simulink model "encoder"  (R2022b)
settings: Solver=VariableStepAuto  StartTime=0.0  StopTime=10.0  RelTol=1e-3
libraries: simulink x1, spsSampleandHoldLib x1
settings Model: Creator=mluser  LastModifiedBy=mluser

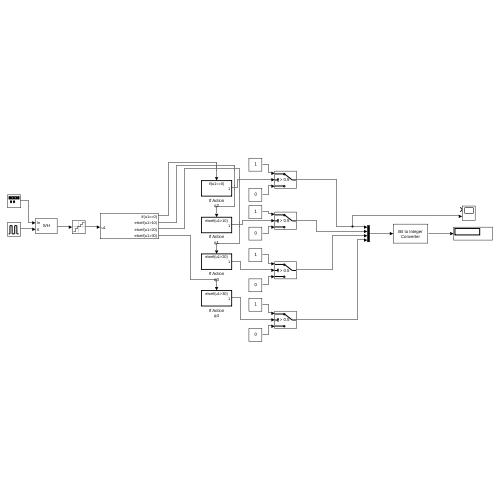
[thumbnail: Simulink's stored preview of the top-level diagram]
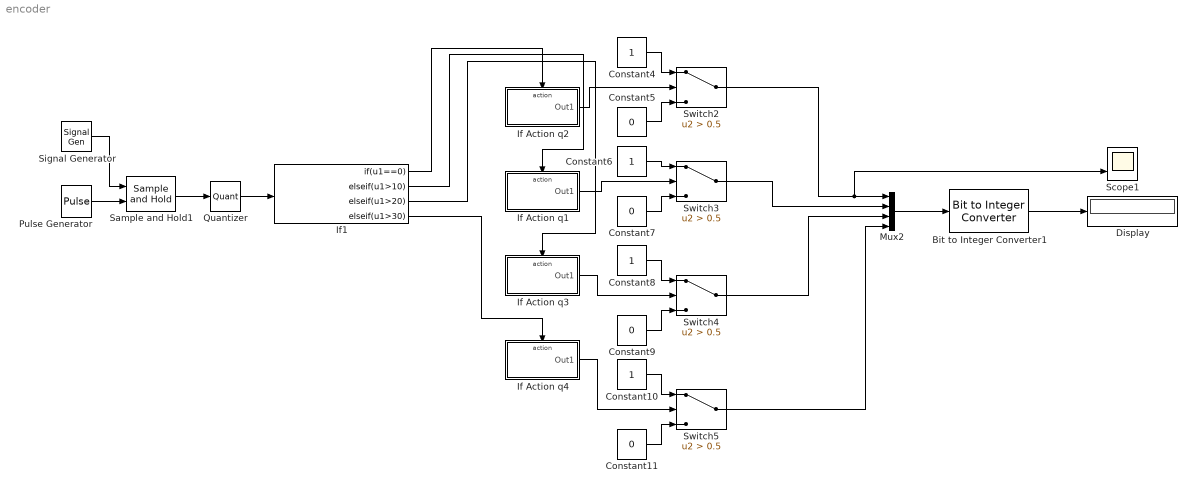
== system encoder ==
  Bit to Integer Converter1 : simulink/Logic and Bit Operations/Bit to Integer Converter  nbits=4  bitOrder=MSB first  signedOutputValues=Unsigned  outDtype=Inherit via internal rule  outDtypeSigned=Inherit via internal rule
  Constant{4,6,8,10} (4 alike) : Constant
  Constant{5,7,9,11} (4 alike) : Constant  Value=0
  Display : Display
  If Action q1 : Subsystem  TreatAsAtomicUnit=on
  If Action q2 : Subsystem  TreatAsAtomicUnit=on
  If Action q3 : Subsystem  TreatAsAtomicUnit=on
  If Action q4 : Subsystem  TreatAsAtomicUnit=on
  If1 : If  IfExpression=u1==0  ElseIfExpressions=u1>10,u1>20,u1>30  ShowElse=off
  Mux2 : Mux
  Pulse Generator : DiscretePulseGenerator  PulseType=Time based  Period=0.1  PulseWidth=5
  Quantizer : Quantizer
  Sample and Hold1 : spsSampleandHoldLib/Sample and Hold  ic=0  Ts=0
      settings: LibrarySourceBlock=|
      | sps_lib/Control/Sample and
      | Hold
  Scope1 : Scope  NumInputPorts=2
  Signal Generator : SignalGenerator  Amplitude=40  Units=rad/sec
  Switch{2..5} (4 alike) : Switch  Criteria=u2 > Threshold  Threshold=0.5  SaturateOnIntegerOverflow=off  InputSameDT=off
  wires:
  Pulse Generator/1 -> Sample and Hold1/2
  Signal Generator/1 -> Sample and Hold1/1
  Bit to Integer Converter1/1 -> Display/1
  If1/1 -> If Action q2/Action
  If1/2 -> If Action q1/Action
  If1/3 -> If Action q3/Action
  Mux2/1 -> Bit to Integer Converter1/1
  If1/4 -> If Action q4/Action
  Switch2/1 -> Scope1/2, Mux2/1
  Constant5/1 -> Switch2/3
  If Action q2/1(Out1) -> Switch2/2
  Constant4/1 -> Switch2/1
  Switch3/1 -> Mux2/2
  Constant6/1 -> Switch3/1
  If Action q1/1(Out1) -> Switch3/2
  Constant7/1 -> Switch3/3
  Switch4/1 -> Mux2/3
  Constant8/1 -> Switch4/1
  If Action q3/1(Out1) -> Switch4/2
  Constant9/1 -> Switch4/3
  Switch5/1 -> Mux2/4
  Constant10/1 -> Switch5/1
  If Action q4/1(Out1) -> Switch5/2
  Constant11/1 -> Switch5/3
  Sample and Hold1/1 -> Quantizer/1
  Quantizer/1 -> If1/1

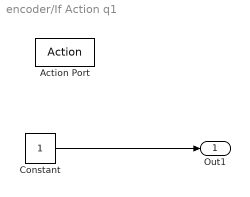
== system encoder/If Action q1 ==
  Action Port : ActionPort  ActionPortLabel=elseif(u1>10)
  Constant : Constant
  Out1 : Outport
  wires:
  Constant/1 -> Out1/1

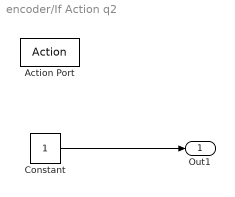
== system encoder/If Action q2 ==
  Action Port : ActionPort  ActionPortLabel=if(u1==0)
  Constant : Constant
  Out1 : Outport
  wires:
  Constant/1 -> Out1/1

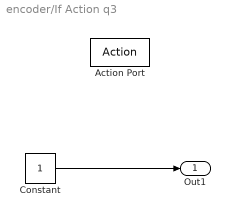
== system encoder/If Action q3 ==
  Action Port : ActionPort  ActionPortLabel=elseif(u1>20)
  Constant : Constant
  Out1 : Outport
  wires:
  Constant/1 -> Out1/1

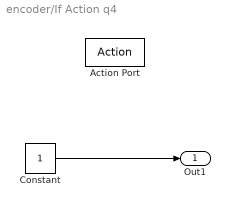
== system encoder/If Action q4 ==
  Action Port : ActionPort  ActionPortLabel=elseif(u1>30)
  Constant : Constant
  Out1 : Outport
  wires:
  Constant/1 -> Out1/1
